simulink model "Tetris"  (R2023a)
settings: Solver=VariableStepAuto  StartTime=0.0  StopTime=inf  RelTol=1e-3  EnableMultiTasking=on
libraries: Miscellaneous x183, Byte_Multiplexers_Lib x77, Tetris_Lib x34, simulink_extras x11, Counters_Lib x7, Arithmetic_Operations_Lib x5, Word_Multiplexers_Lib x5, Decoders_Lib x4, Memory_Blocks_Lib x3, Bit_Multiplexers_Lib x2, dspobslib x1
(part 3 of 3)

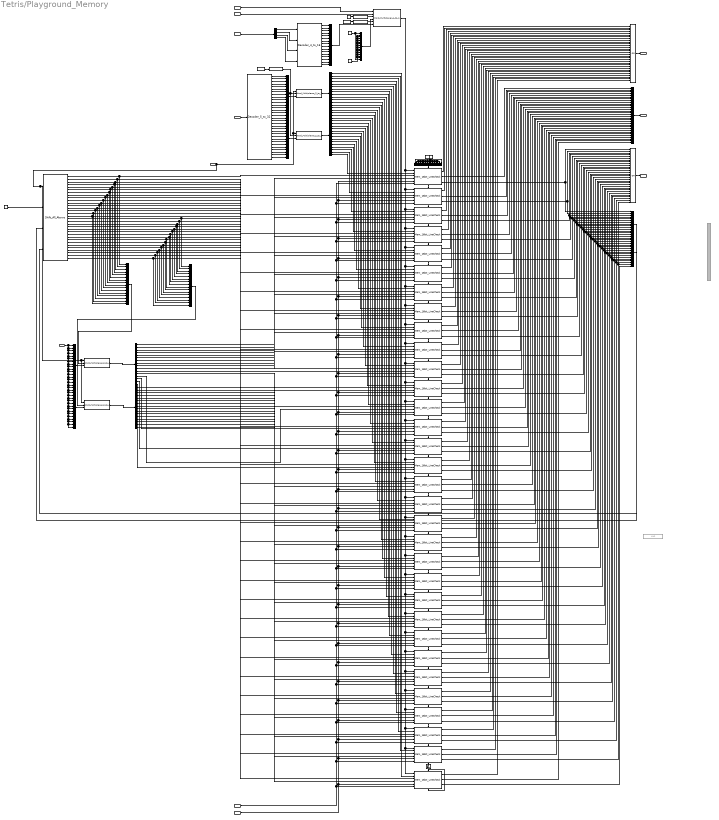
== system Tetris/Playground_Memory ==
  Sel_X(1B) : Inport
  Sel_Y(1B) : Inport  Port=2
  RowAccessUp(1b) : Inport  Port=3
  RowAccessDn(1b) : Inport  Port=4
  Write(1b) : Inport  Port=5
  Shift(1b) : Inport  Port=6
  Data(1b) : Inport  Port=7
  Clk : Inport  Port=8  OutDataTypeStr=boolean
  Bus Creator{1..2,4..6,8..13} (11 alike) : BusCreator  Inputs=16
  Bus Creator3 : BusCreator  Inputs=32
  Bus Creator7 : BusCreator  Commented=on  Inputs=32
  Bus Selector1 : BusSelector  OutputSignals=signal5,signal6,signal7,signal8
  Bus Selector{2..5} (4 alike) : BusSelector  OutputSignals=signal1,signal2,signal3,signal4,signal5,signal6,signal7,signal8,signal9,signal10,signal11,signal12,signal13,signal14,signal15,signal16
  Decoder_4_to_16 : Decoders_Lib/Decoders_Lib/Decoder_4_to_16  SystemSampleTime=-1  VariantActivationTime=update diagram  Latency=0  AutoFrameSizeCalculation=off
  Decoder_5_to_32 : Decoders_Lib/Decoders_Lib/Decoder_5_to_32  SystemSampleTime=-1  VariantActivationTime=update diagram  Latency=0  AutoFrameSizeCalculation=off
  Logical Operator1 : Logic  Operator=OR  Inputs=32  IconShape=distinctive  AllPortsSameDT=off  OutDataTypeStr=boolean
  Logical Operator2 : Logic  Commented=on  Inputs=12  IconShape=distinctive  AllPortsSameDT=off  OutDataTypeStr=boolean
  Logical Operator3 : Logic  Operator=OR  Inputs=31  IconShape=distinctive  AllPortsSameDT=off  OutDataTypeStr=boolean
  Mem_16bit_LineCheck{,1..31} (32 alike) : Tetris_Lib/Mem_16bit_LineCheck  SystemSampleTime=-1  VariantActivationTime=update diagram  Latency=0  AutoFrameSizeCalculation=off
      settings: PortSchema="{\"entries\":[{\"content\":{\"sides\":[{\"content\":{\"connectorIds\":[\"In1\",\"In2\",\"In3\",\"In4\",\"In5\",\"In6\"]},\"type\":\"ConnectorPlacement.EquallySpacedRectSide\",\"uuid\":\"8c2b0956-6f9d-4511-a90f-b568422ac059\"},{\"content\":{\"connectorIds\":[\"Out1\",\"Out2\",\"Out3\"],\"side\":\"RIGHT\"},\"type\":\"ConnectorPlacement.EquallySpacedRectSide\",\"uuid\":\"f2746d35-82bb-4709-925e-ccfde81ba195\"},{\"content\":{\"connectorIds\":[\"In7\"],\"side\":\"TOP\"},\"type\":\"ConnectorPlacement.EquallySpacedRectSide\",\"uuid\":\"2c21dbc3-5fbd-4074-80c1-0ed6354c6907\"},{\"content\":{\"connectorIds\":[\"Out4\"],\"side\":\"BOTTOM\"},\"type\":\"ConnectorPlacement.EquallySpacedRectSide\",\"uuid\":\"e35f839b-c525-4d99-8eb1-36043d411746\"}]},\"type\":\"ConnectorPlacement.EquallySpacedConnector\",\"uuid\":\"65dd92b9-0be0-4546-ad93-b6d7cfee0a19\"}],\"packageUris\":[\"http://schema.mathworks.com/mf0/Connector/R2020b\"],\"version\":\"1.0\"}"
  None1 : Constant  Value=0  OutDataTypeStr=boolean
  None2 : Constant  Value=0  OutDataTypeStr=boolean
  None3 : Constant  Value=0  OutDataTypeStr=boolean
  None4 : Constant  OutDataTypeStr=boolean
  NotUsed : Constant  Value=0  OutDataTypeStr=uint16
  SelectAllColumns : Constant  Value=65535  OutDataTypeStr=uint16
  SelectAllRows : Constant  Value=65535  OutDataTypeStr=uint16
  SelectInnerColumns : Constant  OutDataTypeStr=boolean
  Shift_All_Above : Tetris_Lib/Shift_All_Above  SystemSampleTime=-1  VariantActivationTime=update diagram  Latency=0  AutoFrameSizeCalculation=off
  Terminator : Terminator
  Word_Multiplexer_2_to_{1..4} (4 alike) : Word_Multiplexers_Lib/Word_Multiplexers_Lib/Word_Multiplexer_2_to_1  SystemSampleTime=-1  VariantActivationTime=update diagram  Latency=0  AutoFrameSizeCalculation=off
  Word_Multiplexer_4_to_1 : Word_Multiplexers_Lib/Word_Multiplexers_Lib/Word_Multiplexer_4_to_1  SystemSampleTime=-1  VariantActivationTime=update diagram  Latency=0  AutoFrameSizeCalculation=off
  uint_to_bus : Miscellaneous/uint_to_bus  SystemSampleTime=-1  VariantActivationTime=update diagram  Latency=0  AutoFrameSizeCalculation=off
  uint_to_bus1 : Miscellaneous/uint_to_bus  SystemSampleTime=-1  VariantActivationTime=update diagram  Latency=0  AutoFrameSizeCalculation=off
  uint_to_bus2 : Miscellaneous/uint_to_bus  SystemSampleTime=-1  VariantActivationTime=update diagram  Latency=0  AutoFrameSizeCalculation=off
  Video(32x16b) : Outport
  PixelOut(1b) : Outport  Port=2
  LineDone(1b) : Outport  Port=3
  wires:
  Bus Selector1/1 -> Decoder_4_to_16/1  "<signal5>"
  Bus Selector1/2 -> Decoder_4_to_16/2  "<signal6>"
  Bus Selector1/3 -> Decoder_4_to_16/3  "<signal7>"
  Bus Selector1/4 -> Decoder_4_to_16/4  "<signal8>"
  Sel_X(1B)/1 -> Bus Selector1/1
  Sel_Y(1B)/1 -> Decoder_5_to_32/1
  Bus Selector3/16 -> Mem_16bit_LineCheck31/2  "<signal16>"
  Bus Selector3/15 -> Mem_16bit_LineCheck30/2  "<signal15>"
  Bus Selector3/14 -> Mem_16bit_LineCheck29/2  "<signal14>"
  Bus Selector3/13 -> Mem_16bit_LineCheck28/2  "<signal13>"
  Bus Selector3/12 -> Mem_16bit_LineCheck27/2  "<signal12>"
  Bus Selector3/11 -> Mem_16bit_LineCheck26/2  "<signal11>"
  Bus Selector3/10 -> Mem_16bit_LineCheck25/2  "<signal10>"
  Bus Selector3/9 -> Mem_16bit_LineCheck24/2  "<signal9>"
  Bus Selector3/8 -> Mem_16bit_LineCheck23/2  "<signal8>"
  Bus Selector3/7 -> Mem_16bit_LineCheck22/2  "<signal7>"
  Bus Selector3/6 -> Mem_16bit_LineCheck21/2  "<signal6>"
  Bus Selector3/5 -> Mem_16bit_LineCheck20/2  "<signal5>"
  Bus Selector3/4 -> Mem_16bit_LineCheck19/2  "<signal4>"
  Bus Selector3/3 -> Mem_16bit_LineCheck18/2  "<signal3>"
  Bus Selector3/2 -> Mem_16bit_LineCheck17/2  "<signal2>"
  Bus Selector3/1 -> Mem_16bit_LineCheck16/2  "<signal1>"
  Bus Selector2/16 -> Mem_16bit_LineCheck15/2  "<signal16>"
  Bus Selector2/15 -> Mem_16bit_LineCheck14/2  "<signal15>"
  Bus Selector2/14 -> Mem_16bit_LineCheck13/2  "<signal14>"
  Bus Selector2/13 -> Mem_16bit_LineCheck12/2  "<signal13>"
  Bus Selector2/12 -> Mem_16bit_LineCheck11/2  "<signal12>"
  Bus Selector2/11 -> Mem_16bit_LineCheck10/2  "<signal11>"
  Bus Selector2/10 -> Mem_16bit_LineCheck9/2  "<signal10>"
  Bus Selector2/9 -> Mem_16bit_LineCheck8/2  "<signal9>"
  Bus Selector2/8 -> Mem_16bit_LineCheck7/2  "<signal8>"
  Bus Selector2/7 -> Mem_16bit_LineCheck6/2  "<signal7>"
  Bus Selector2/6 -> Mem_16bit_LineCheck5/2  "<signal6>"
  Bus Selector2/5 -> Mem_16bit_LineCheck4/2  "<signal5>"
  Bus Selector2/4 -> Mem_16bit_LineCheck3/2  "<signal4>"
  Bus Selector2/3 -> Mem_16bit_LineCheck2/2  "<signal3>"
  Bus Selector2/2 -> Mem_16bit_LineCheck1/2  "<signal2>"
  Bus Selector2/1 -> Mem_16bit_LineCheck/2  "<signal1>"
  Data(1b)/1 -> Mem_16bit_LineCheck31/5, Mem_16bit_LineCheck30/5, Mem_16bit_LineCheck29/5, Mem_16bit_LineCheck28/5, Mem_16bit_LineCheck27/5, Mem_16bit_LineCheck26/5, Mem_16bit_LineCheck25/5, Mem_16bit_LineCheck24/5, Mem_16bit_LineCheck23/5, Mem_16bit_LineCheck22/5, Mem_16bit_LineCheck21/5, Mem_16bit_LineCheck20/5, Mem_16bit_LineCheck19/5, Mem_16bit_LineCheck18/5, Mem_16bit_LineCheck17/5, Mem_16bit_LineCheck16/5, Mem_16bit_LineCheck15/5, Mem_16bit_LineCheck14/5, Mem_16bit_LineCheck13/5, Mem_16bit_LineCheck12/5, Mem_16bit_LineCheck11/5, Mem_16bit_LineCheck10/5, Mem_16bit_LineCheck9/5, Mem_16bit_LineCheck8/5, Mem_16bit_LineCheck7/5, Mem_16bit_LineCheck6/5, Mem_16bit_LineCheck5/5, Mem_16bit_LineCheck4/5, Mem_16bit_LineCheck3/5, Mem_16bit_LineCheck2/5, Mem_16bit_LineCheck1/5, Mem_16bit_LineCheck/5
  Clk/1 -> Mem_16bit_LineCheck31/6, Mem_16bit_LineCheck30/6, Mem_16bit_LineCheck29/6, Mem_16bit_LineCheck28/6, Mem_16bit_LineCheck27/6, Mem_16bit_LineCheck26/6, Mem_16bit_LineCheck25/6, Mem_16bit_LineCheck24/6, Mem_16bit_LineCheck23/6, Mem_16bit_LineCheck22/6, Mem_16bit_LineCheck21/6, Mem_16bit_LineCheck20/6, Mem_16bit_LineCheck19/6, Mem_16bit_LineCheck18/6, Mem_16bit_LineCheck17/6, Mem_16bit_LineCheck16/6, Mem_16bit_LineCheck15/6, Mem_16bit_LineCheck14/6, Mem_16bit_LineCheck13/6, Mem_16bit_LineCheck12/6, Mem_16bit_LineCheck11/6, Mem_16bit_LineCheck10/6, Mem_16bit_LineCheck9/6, Mem_16bit_LineCheck8/6, Mem_16bit_LineCheck7/6, Mem_16bit_LineCheck6/6, Mem_16bit_LineCheck5/6, Mem_16bit_LineCheck4/6, Mem_16bit_LineCheck3/6, Mem_16bit_LineCheck2/6, Mem_16bit_LineCheck1/6, Mem_16bit_LineCheck/6
  Mem_16bit_LineCheck31/2 -> Bus Creator3/1
  Mem_16bit_LineCheck30/2 -> Bus Creator3/2
  Mem_16bit_LineCheck29/2 -> Bus Creator3/3
  Mem_16bit_LineCheck28/2 -> Bus Creator3/4
  Mem_16bit_LineCheck27/2 -> Bus Creator3/5
  Mem_16bit_LineCheck26/2 -> Bus Creator3/6
  Mem_16bit_LineCheck25/2 -> Bus Creator3/7
  Mem_16bit_LineCheck24/2 -> Bus Creator3/8
  Mem_16bit_LineCheck23/2 -> Bus Creator3/9
  Mem_16bit_LineCheck22/2 -> Bus Creator3/10
  Mem_16bit_LineCheck21/2 -> Bus Creator3/11
  Mem_16bit_LineCheck20/2 -> Bus Creator3/12
  Mem_16bit_LineCheck19/2 -> Bus Creator3/13
  Mem_16bit_LineCheck18/2 -> Bus Creator3/14
  Mem_16bit_LineCheck17/2 -> Bus Creator3/15
  Mem_16bit_LineCheck16/2 -> Bus Creator3/16
  Mem_16bit_LineCheck15/2 -> Bus Creator3/17
  Mem_16bit_LineCheck14/2 -> Bus Creator3/18
  Mem_16bit_LineCheck13/2 -> Bus Creator3/19
  Mem_16bit_LineCheck12/2 -> Bus Creator3/20
  Mem_16bit_LineCheck11/2 -> Bus Creator3/21
  Mem_16bit_LineCheck10/2 -> Bus Creator3/22
  Mem_16bit_LineCheck9/2 -> Bus Creator3/23
  Mem_16bit_LineCheck8/2 -> Bus Creator3/24
  Mem_16bit_LineCheck7/2 -> Bus Creator3/25
  Mem_16bit_LineCheck6/2 -> Bus Creator3/26
  Mem_16bit_LineCheck5/2 -> Bus Creator3/27
  Mem_16bit_LineCheck4/2 -> Bus Creator3/28
  Mem_16bit_LineCheck3/2 -> Bus Creator3/29
  Mem_16bit_LineCheck2/2 -> Bus Creator3/30
  Mem_16bit_LineCheck1/2 -> Bus Creator3/31
  Mem_16bit_LineCheck/2 -> Bus Creator3/32
  Mem_16bit_LineCheck31/1 -> Logical Operator1/1
  Mem_16bit_LineCheck30/1 -> Logical Operator1/2
  Mem_16bit_LineCheck29/1 -> Logical Operator1/3
  Mem_16bit_LineCheck28/1 -> Logical Operator1/4
  Mem_16bit_LineCheck27/1 -> Logical Operator1/5
  Mem_16bit_LineCheck26/1 -> Logical Operator1/6
  Mem_16bit_LineCheck25/1 -> Logical Operator1/7
  Mem_16bit_LineCheck24/1 -> Logical Operator1/8
  Mem_16bit_LineCheck23/1 -> Logical Operator1/9
  Mem_16bit_LineCheck22/1 -> Logical Operator1/10
  Mem_16bit_LineCheck21/1 -> Logical Operator1/11
  Mem_16bit_LineCheck20/1 -> Logical Operator1/12
  Mem_16bit_LineCheck19/1 -> Logical Operator1/13
  Mem_16bit_LineCheck18/1 -> Logical Operator1/14
  Mem_16bit_LineCheck17/1 -> Logical Operator1/15
  Mem_16bit_LineCheck16/1 -> Logical Operator1/16
  Mem_16bit_LineCheck15/1 -> Logical Operator1/17
  Mem_16bit_LineCheck14/1 -> Logical Operator1/18
  Mem_16bit_LineCheck13/1 -> Logical Operator1/19
  Mem_16bit_LineCheck12/1 -> Logical Operator1/20
  Mem_16bit_LineCheck11/1 -> Logical Operator1/21
  Mem_16bit_LineCheck10/1 -> Logical Operator1/22
  Mem_16bit_LineCheck9/1 -> Logical Operator1/23
  Mem_16bit_LineCheck8/1 -> Logical Operator1/24
  Mem_16bit_LineCheck7/1 -> Logical Operator1/25
  Mem_16bit_LineCheck6/1 -> Logical Operator1/26
  Mem_16bit_LineCheck5/1 -> Logical Operator1/27
  Mem_16bit_LineCheck4/1 -> Logical Operator1/28
  Mem_16bit_LineCheck3/1 -> Logical Operator1/29
  Mem_16bit_LineCheck2/1 -> Logical Operator1/30
  Mem_16bit_LineCheck1/1 -> Logical Operator1/31
  Mem_16bit_LineCheck/1 -> Logical Operator1/32
  Bus Creator3/1 -> Video(32x16b)/1
  Logical Operator1/1 -> PixelOut(1b)/1
  RowAccessUp(1b)/1 -> Word_Multiplexer_4_to_1/2
  Bus Creator1/1 -> Word_Multiplexer_4_to_1/6
  Decoder_4_to_16/1 -> Bus Creator1/1
  Decoder_4_to_16/2 -> Bus Creator1/2
  Decoder_4_to_16/3 -> Bus Creator1/3
  Decoder_4_to_16/4 -> Bus Creator1/4
  Decoder_4_to_16/5 -> Bus Creator1/5
  Decoder_4_to_16/6 -> Bus Creator1/6
  Decoder_4_to_16/7 -> Bus Creator1/7
  Decoder_4_to_16/8 -> Bus Creator1/8
  Decoder_4_to_16/9 -> Bus Creator1/9
  Decoder_4_to_16/10 -> Bus Creator1/10
  Decoder_4_to_16/11 -> Bus Creator1/11
  Decoder_4_to_16/12 -> Bus Creator1/12
  Decoder_4_to_16/13 -> Bus Creator1/13
  Decoder_4_to_16/14 -> Bus Creator1/14
  Decoder_4_to_16/15 -> Bus Creator1/15
  Decoder_4_to_16/16 -> Bus Creator1/16
  Word_Multiplexer_4_to_1/1 -> Mem_16bit_LineCheck/1, Mem_16bit_LineCheck1/1, Mem_16bit_LineCheck2/1, Mem_16bit_LineCheck3/1, Mem_16bit_LineCheck4/1, Mem_16bit_LineCheck5/1, Mem_16bit_LineCheck6/1, Mem_16bit_LineCheck7/1, Mem_16bit_LineCheck8/1, Mem_16bit_LineCheck9/1, Mem_16bit_LineCheck10/1, Mem_16bit_LineCheck11/1, Mem_16bit_LineCheck12/1, Mem_16bit_LineCheck13/1, Mem_16bit_LineCheck14/1, Mem_16bit_LineCheck15/1, Mem_16bit_LineCheck16/1, Mem_16bit_LineCheck17/1, Mem_16bit_LineCheck18/1, Mem_16bit_LineCheck19/1, Mem_16bit_LineCheck20/1, Mem_16bit_LineCheck21/1, Mem_16bit_LineCheck22/1, Mem_16bit_LineCheck23/1, Mem_16bit_LineCheck24/1, Mem_16bit_LineCheck25/1, Mem_16bit_LineCheck26/1, Mem_16bit_LineCheck27/1, Mem_16bit_LineCheck28/1, Mem_16bit_LineCheck29/1, Mem_16bit_LineCheck30/1, Mem_16bit_LineCheck31/1
  Mem_16bit_LineCheck2/4 -> Mem_16bit_LineCheck1/7
  Mem_16bit_LineCheck1/4 -> Terminator/1
  Bus Creator2/1 -> Mem_16bit_LineCheck31/7
  Mem_16bit_LineCheck/4 -> Mem_16bit_LineCheck/7
  SelectInnerColumns/1 -> Bus Creator4/2, Bus Creator4/3, Bus Creator4/4, Bus Creator4/5, Bus Creator4/6, Bus Creator4/7, Bus Creator4/8, Bus Creator4/9, Bus Creator4/10, Bus Creator4/11, Bus Creator4/12, Bus Creator4/13, Bus Creator4/14, Bus Creator4/15
  None3/1 -> Bus Creator4/16, Bus Creator4/1
  Bus Creator4/1 -> Word_Multiplexer_4_to_1/4
  RowAccessDn(1b)/1 -> Word_Multiplexer_4_to_1/1
  uint_to_bus/1 -> Word_Multiplexer_4_to_1/3
  NotUsed/1 -> uint_to_bus/1
  SelectAllColumns/1 -> uint_to_bus1/1
  uint_to_bus1/1 -> Word_Multiplexer_4_to_1/5
  None4/1 -> Bus Creator2/16, Bus Creator2/1
  Decoder_5_to_32/18 -> Bus Creator5/2
  Decoder_5_to_32/19 -> Bus Creator5/3
  Decoder_5_to_32/20 -> Bus Creator5/4
  Decoder_5_to_32/21 -> Bus Creator5/5
  Decoder_5_to_32/22 -> Bus Creator5/6
  Decoder_5_to_32/23 -> Bus Creator5/7
  Decoder_5_to_32/24 -> Bus Creator5/8
  Decoder_5_to_32/25 -> Bus Creator5/9
  Decoder_5_to_32/26 -> Bus Creator5/10
  Decoder_5_to_32/27 -> Bus Creator5/11
  Decoder_5_to_32/28 -> Bus Creator5/12
  Decoder_5_to_32/29 -> Bus Creator5/13
  Decoder_5_to_32/30 -> Bus Creator5/14
  Decoder_5_to_32/31 -> Bus Creator5/15
  Decoder_5_to_32/32 -> Bus Creator5/16
  Decoder_5_to_32/1 -> Bus Creator6/1
  Decoder_5_to_32/2 -> Bus Creator6/2
  Decoder_5_to_32/3 -> Bus Creator6/3
  Decoder_5_to_32/4 -> Bus Creator6/4
  Decoder_5_to_32/5 -> Bus Creator6/5
  Decoder_5_to_32/6 -> Bus Creator6/6
  Decoder_5_to_32/7 -> Bus Creator6/7
  Decoder_5_to_32/8 -> Bus Creator6/8
  Decoder_5_to_32/9 -> Bus Creator6/9
  Decoder_5_to_32/10 -> Bus Creator6/10
  Decoder_5_to_32/11 -> Bus Creator6/11
  Decoder_5_to_32/12 -> Bus Creator6/12
  Decoder_5_to_32/13 -> Bus Creator6/13
  Decoder_5_to_32/14 -> Bus Creator6/14
  Decoder_5_to_32/15 -> Bus Creator6/15
  Decoder_5_to_32/16 -> Bus Creator6/16
  Decoder_5_to_32/17 -> Bus Creator5/1
  Bus Creator6/1 -> Word_Multiplexer_2_to_1/3
  Bus Creator5/1 -> Word_Multiplexer_2_to_2/3
  Word_Multiplexer_2_to_1/1 -> Bus Selector2/1
  Word_Multiplexer_2_to_2/1 -> Bus Selector3/1
  uint_to_bus2/1 -> Word_Multiplexer_2_to_2/2, Word_Multiplexer_2_to_1/2
  SelectAllRows/1 -> uint_to_bus2/1
  Mem_16bit_LineCheck4/4 -> Mem_16bit_LineCheck3/7
  Mem_16bit_LineCheck5/4 -> Mem_16bit_LineCheck4/7
  Mem_16bit_LineCheck6/4 -> Mem_16bit_LineCheck5/7
  Mem_16bit_LineCheck7/4 -> Mem_16bit_LineCheck6/7
  Mem_16bit_LineCheck8/4 -> Mem_16bit_LineCheck7/7
  Mem_16bit_LineCheck9/4 -> Mem_16bit_LineCheck8/7
  Mem_16bit_LineCheck10/4 -> Mem_16bit_LineCheck9/7
  Mem_16bit_LineCheck11/4 -> Mem_16bit_LineCheck10/7
  Mem_16bit_LineCheck12/4 -> Mem_16bit_LineCheck11/7
  Mem_16bit_LineCheck13/4 -> Mem_16bit_LineCheck12/7
  Mem_16bit_LineCheck14/4 -> Mem_16bit_LineCheck13/7
  Mem_16bit_LineCheck15/4 -> Mem_16bit_LineCheck14/7
  Mem_16bit_LineCheck16/4 -> Mem_16bit_LineCheck15/7
  Mem_16bit_LineCheck17/4 -> Mem_16bit_LineCheck16/7
  Mem_16bit_LineCheck18/4 -> Mem_16bit_LineCheck17/7
  Mem_16bit_LineCheck19/4 -> Mem_16bit_LineCheck18/7
  Mem_16bit_LineCheck20/4 -> Mem_16bit_LineCheck19/7
  Mem_16bit_LineCheck21/4 -> Mem_16bit_LineCheck20/7
  Mem_16bit_LineCheck22/4 -> Mem_16bit_LineCheck21/7
  Mem_16bit_LineCheck23/4 -> Mem_16bit_LineCheck22/7
  Mem_16bit_LineCheck24/4 -> Mem_16bit_LineCheck23/7
  Mem_16bit_LineCheck25/4 -> Mem_16bit_LineCheck24/7
  Mem_16bit_LineCheck26/4 -> Mem_16bit_LineCheck25/7
  Mem_16bit_LineCheck27/4 -> Mem_16bit_LineCheck26/7
  Mem_16bit_LineCheck28/4 -> Mem_16bit_LineCheck27/7
  Mem_16bit_LineCheck29/4 -> Mem_16bit_LineCheck28/7
  Mem_16bit_LineCheck30/4 -> Mem_16bit_LineCheck29/7
  Mem_16bit_LineCheck31/4 -> Mem_16bit_LineCheck30/7
  Mem_16bit_LineCheck3/4 -> Mem_16bit_LineCheck2/7
  Mem_16bit_LineCheck31/3 -> Bus Creator10/1, Logical Operator3/1
  Mem_16bit_LineCheck30/3 -> Bus Creator10/2, Logical Operator3/2
  Mem_16bit_LineCheck29/3 -> Bus Creator10/3, Logical Operator3/3
  Mem_16bit_LineCheck28/3 -> Bus Creator10/4, Logical Operator3/4
  Mem_16bit_LineCheck27/3 -> Bus Creator10/5, Logical Operator3/5
  Mem_16bit_LineCheck26/3 -> Bus Creator10/6, Logical Operator3/6
  Mem_16bit_LineCheck25/3 -> Bus Creator10/7, Logical Operator3/7
  Mem_16bit_LineCheck24/3 -> Bus Creator10/8, Logical Operator3/8
  Mem_16bit_LineCheck22/3 -> Bus Creator10/10, Logical Operator3/10
  Mem_16bit_LineCheck21/3 -> Bus Creator10/11, Logical Operator3/11
  Mem_16bit_LineCheck20/3 -> Bus Creator10/12, Logical Operator3/12
  Mem_16bit_LineCheck19/3 -> Bus Creator10/13, Logical Operator3/13
  Mem_16bit_LineCheck18/3 -> Bus Creator10/14, Logical Operator3/14
  Mem_16bit_LineCheck17/3 -> Bus Creator10/15, Logical Operator3/15
  Mem_16bit_LineCheck16/3 -> Bus Creator10/16, Logical Operator3/16
  Mem_16bit_LineCheck15/3 -> Bus Creator11/1, Logical Operator3/17
  Mem_16bit_LineCheck14/3 -> Bus Creator11/2, Logical Operator3/18
  Mem_16bit_LineCheck13/3 -> Bus Creator11/3, Logical Operator3/19
  Mem_16bit_LineCheck12/3 -> Bus Creator11/4, Logical Operator3/20
  Mem_16bit_LineCheck11/3 -> Bus Creator11/5, Logical Operator3/21
  Mem_16bit_LineCheck10/3 -> Bus Creator11/6, Logical Operator3/22
  Mem_16bit_LineCheck9/3 -> Bus Creator11/7, Logical Operator3/23
  Mem_16bit_LineCheck8/3 -> Bus Creator11/8, Logical Operator3/24
  Mem_16bit_LineCheck7/3 -> Bus Creator11/9, Logical Operator3/25
  Mem_16bit_LineCheck6/3 -> Bus Creator11/10, Logical Operator3/26
  Mem_16bit_LineCheck5/3 -> Bus Creator11/11, Logical Operator3/27
  Mem_16bit_LineCheck4/3 -> Bus Creator11/12, Logical Operator3/28
  Mem_16bit_LineCheck3/3 -> Bus Creator11/13, Logical Operator3/29
  Mem_16bit_LineCheck2/3 -> Bus Creator11/14, Logical Operator3/30
  Mem_16bit_LineCheck1/3 -> Bus Creator11/15, Logical Operator3/31
  Bus Creator10/1 -> Shift_All_Above/3
  Shift_All_Above/1 -> Bus Creator12/1, Mem_16bit_LineCheck31/3
  Shift_All_Above/2 -> Bus Creator12/2, Mem_16bit_LineCheck30/3
  Shift_All_Above/3 -> Bus Creator12/3, Mem_16bit_LineCheck29/3
  Shift_All_Above/4 -> Bus Creator12/4, Mem_16bit_LineCheck28/3
  Shift_All_Above/5 -> Bus Creator12/5, Mem_16bit_LineCheck27/3
  Shift_All_Above/6 -> Bus Creator12/6, Mem_16bit_LineCheck26/3
  Shift_All_Above/7 -> Bus Creator12/7, Mem_16bit_LineCheck25/3
  Shift_All_Above/8 -> Bus Creator12/8, Mem_16bit_LineCheck24/3
  Shift_All_Above/9 -> Bus Creator12/9, Mem_16bit_LineCheck23/3
  Shift_All_Above/10 -> Bus Creator12/10, Mem_16bit_LineCheck22/3
  Shift_All_Above/11 -> Bus Creator12/11, Mem_16bit_LineCheck21/3
  Shift_All_Above/12 -> Bus Creator12/12, Mem_16bit_LineCheck20/3
  Shift_All_Above/13 -> Bus Creator12/13, Mem_16bit_LineCheck19/3
  Shift_All_Above/14 -> Bus Creator12/14, Mem_16bit_LineCheck18/3
  Shift_All_Above/15 -> Bus Creator12/15, Mem_16bit_LineCheck17/3
  Shift_All_Above/16 -> Bus Creator12/16, Mem_16bit_LineCheck16/3
  Shift_All_Above/17 -> Bus Creator13/1, Mem_16bit_LineCheck15/3
  Shift_All_Above/18 -> Bus Creator13/2, Mem_16bit_LineCheck14/3
  Shift_All_Above/19 -> Bus Creator13/3, Mem_16bit_LineCheck13/3
  Shift_All_Above/20 -> Bus Creator13/4, Mem_16bit_LineCheck12/3
  Shift_All_Above/21 -> Bus Creator13/5, Mem_16bit_LineCheck11/3
  Shift_All_Above/22 -> Bus Creator13/6, Mem_16bit_LineCheck10/3
  Shift_All_Above/23 -> Bus Creator13/7, Mem_16bit_LineCheck9/3
  Shift_All_Above/24 -> Bus Creator13/8, Mem_16bit_LineCheck8/3
  Shift_All_Above/25 -> Bus Creator13/9, Mem_16bit_LineCheck7/3
  Shift_All_Above/26 -> Bus Creator13/10, Mem_16bit_LineCheck6/3
  Shift_All_Above/27 -> Bus Creator13/11, Mem_16bit_LineCheck5/3
  Shift_All_Above/28 -> Bus Creator13/12, Mem_16bit_LineCheck4/3
  Shift_All_Above/29 -> Bus Creator13/13, Mem_16bit_LineCheck3/3
  Shift_All_Above/30 -> Bus Creator13/14, Mem_16bit_LineCheck2/3
  Shift_All_Above/31 -> Bus Creator13/15, Mem_16bit_LineCheck1/3
  Shift(1b)/1 -> Shift_All_Above/1, Word_Multiplexer_2_to_3/1, Word_Multiplexer_2_to_4/1, Word_Multiplexer_2_to_2/1, Word_Multiplexer_2_to_1/1
  Mem_16bit_LineCheck23/3 -> Bus Creator10/9, Logical Operator3/9
  Logical Operator3/1 -> LineDone(1b)/1
  Mem_16bit_LineCheck/3 -> Bus Creator11/16
  Shift_All_Above/32 -> Bus Creator13/16, Mem_16bit_LineCheck/3
  Bus Creator8/1 -> Word_Multiplexer_2_to_3/3
  Word_Multiplexer_2_to_3/1 -> Bus Selector4/1
  Bus Creator9/1 -> Word_Multiplexer_2_to_4/3
  Word_Multiplexer_2_to_4/1 -> Bus Selector5/1
  Write(1b)/1 -> Bus Creator8/2, Bus Creator8/3, Bus Creator8/4, Bus Creator8/5, Bus Creator8/6, Bus Creator8/7, Bus Creator8/8, Bus Creator8/9, Bus Creator8/10, Bus Creator8/11, Bus Creator8/12, Bus Creator8/13, Bus Creator8/14, Bus Creator8/15, Bus Creator8/16, Bus Creator9/1, Bus Creator9/2, Bus Creator9/3, Bus Creator9/4, Bus Creator9/5, Bus Creator9/6, Bus Creator9/7, Bus Creator9/8, Bus Creator9/9, Bus Creator9/10, Bus Creator9/11, Bus Creator9/12, Bus Creator9/13, Bus Creator9/14, Bus Creator9/15, Bus Creator9/16, Bus Creator8/1
  Bus Selector4/1 -> Mem_16bit_LineCheck31/4  "<signal1>"
  Bus Selector4/2 -> Mem_16bit_LineCheck30/4  "<signal2>"
  Bus Selector4/3 -> Mem_16bit_LineCheck29/4  "<signal3>"
  Bus Selector4/4 -> Mem_16bit_LineCheck28/4  "<signal4>"
  Bus Selector4/5 -> Mem_16bit_LineCheck27/4  "<signal5>"
  Bus Selector4/6 -> Mem_16bit_LineCheck26/4  "<signal6>"
  Bus Selector4/7 -> Mem_16bit_LineCheck25/4  "<signal7>"
  Bus Selector4/8 -> Mem_16bit_LineCheck24/4  "<signal8>"
  Bus Selector4/9 -> Mem_16bit_LineCheck23/4  "<signal9>"
  Bus Selector4/10 -> Mem_16bit_LineCheck22/4  "<signal10>"
  Bus Selector4/11 -> Mem_16bit_LineCheck21/4  "<signal11>"
  Bus Selector4/12 -> Mem_16bit_LineCheck20/4  "<signal12>"
  Bus Selector4/13 -> Mem_16bit_LineCheck19/4  "<signal13>"
  Bus Selector4/14 -> Mem_16bit_LineCheck18/4  "<signal14>"
  Bus Selector4/15 -> Mem_16bit_LineCheck17/4  "<signal15>"
  Bus Selector4/16 -> Mem_16bit_LineCheck16/4  "<signal16>"
  Bus Selector5/1 -> Mem_16bit_LineCheck15/4  "<signal1>"
  Bus Selector5/2 -> Mem_16bit_LineCheck14/4  "<signal2>"
  Bus Selector5/3 -> Mem_16bit_LineCheck13/4  "<signal3>"
  Bus Selector5/4 -> Mem_16bit_LineCheck12/4  "<signal4>"
  Bus Selector5/5 -> Mem_16bit_LineCheck11/4  "<signal5>"
  Bus Selector5/6 -> Mem_16bit_LineCheck10/4  "<signal6>"
  Bus Selector5/7 -> Mem_16bit_LineCheck9/4  "<signal7>"
  Bus Selector5/8 -> Mem_16bit_LineCheck8/4  "<signal8>"
  Bus Selector5/9 -> Mem_16bit_LineCheck7/4  "<signal9>"
  Bus Selector5/10 -> Mem_16bit_LineCheck6/4  "<signal10>"
  Bus Selector5/11 -> Mem_16bit_LineCheck5/4  "<signal11>"
  Bus Selector5/12 -> Mem_16bit_LineCheck4/4  "<signal12>"
  Bus Selector5/13 -> Mem_16bit_LineCheck3/4  "<signal13>"
  Bus Selector5/14 -> Mem_16bit_LineCheck2/4  "<signal14>"
  Bus Selector5/15 -> Mem_16bit_LineCheck1/4  "<signal15>"
  Bus Selector5/16 -> Mem_16bit_LineCheck/4  "<signal16>"
  Bus Creator11/1 -> Shift_All_Above/4
  None2/1 -> Shift_All_Above/2
  Bus Creator12/1 -> Word_Multiplexer_2_to_3/2
  Bus Creator13/1 -> Word_Multiplexer_2_to_4/2
  None1/1 -> Bus Creator2/12, Bus Creator2/14, Bus Creator2/15, Bus Creator2/13, Bus Creator2/11, Bus Creator2/10, Bus Creator2/9, Bus Creator2/2, Bus Creator2/3, Bus Creator2/4, Bus Creator2/5, Bus Creator2/6, Bus Creator2/7, Bus Creator2/8

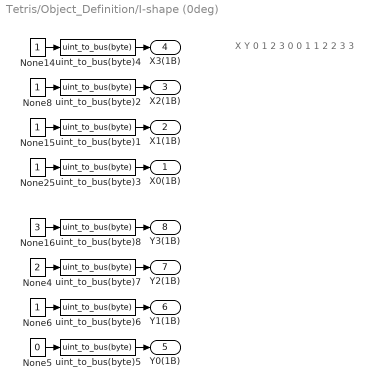
== system Tetris/Object_Definition/I-shape (0deg) ==
  note: X
      |
      | Y
      |
      | 0
      | 1
      | 2
      | 3
      |
      | 0
      |
      | 0
      |
      | 1
      |
      | 1
      |
      | 2
      |
      | 2
      |
      | 3
      |
      | 3
  None{6,8,14..15,25} (5 alike) : Constant  OutDataTypeStr=uint8
  None16 : Constant  Value=3  OutDataTypeStr=uint8
  None4 : Constant  Value=2  OutDataTypeStr=uint8
  None5 : Constant  Value=0  OutDataTypeStr=uint8
  uint_to_bus(byte){1..8} (8 alike) : Miscellaneous/uint_to_bus(byte)  SystemSampleTime=-1  VariantActivationTime=update diagram  Latency=0  AutoFrameSizeCalculation=off
  X0(1B) : Outport
  X1(1B) : Outport  Port=2
  X2(1B) : Outport  Port=3
  X3(1B) : Outport  Port=4
  Y0(1B) : Outport  Port=5
  Y1(1B) : Outport  Port=6
  Y2(1B) : Outport  Port=7
  Y3(1B) : Outport  Port=8
  wires:
  uint_to_bus(byte)4/1 -> X3(1B)/1
  None14/1 -> uint_to_bus(byte)4/1
  None25/1 -> uint_to_bus(byte)3/1
  None8/1 -> uint_to_bus(byte)2/1
  None15/1 -> uint_to_bus(byte)1/1
  uint_to_bus(byte)8/1 -> Y3(1B)/1
  uint_to_bus(byte)6/1 -> Y1(1B)/1
  None6/1 -> uint_to_bus(byte)6/1
  uint_to_bus(byte)7/1 -> Y2(1B)/1
  uint_to_bus(byte)5/1 -> Y0(1B)/1
  None16/1 -> uint_to_bus(byte)8/1
  None5/1 -> uint_to_bus(byte)5/1
  uint_to_bus(byte)1/1 -> X1(1B)/1
  uint_to_bus(byte)3/1 -> X0(1B)/1
  uint_to_bus(byte)2/1 -> X2(1B)/1
  None4/1 -> uint_to_bus(byte)7/1

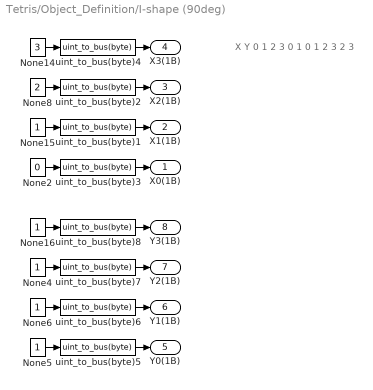
== system Tetris/Object_Definition/I-shape (90deg) ==
  note: X
      |
      | Y
      |
      | 0
      | 1
      | 2
      | 3
      |
      | 0
      |
      | 1
      | 0
      | 1
      | 2
      | 3
      |
      | 2
      |
      | 3
  None14 : Constant  Value=3  OutDataTypeStr=uint8
  None{4..6,15..16} (5 alike) : Constant  OutDataTypeStr=uint8
  None2 : Constant  Value=0  OutDataTypeStr=uint8
  None8 : Constant  Value=2  OutDataTypeStr=uint8
  uint_to_bus(byte){1..8} (8 alike) : Miscellaneous/uint_to_bus(byte)  SystemSampleTime=-1  VariantActivationTime=update diagram  Latency=0  AutoFrameSizeCalculation=off
  X0(1B) : Outport
  X1(1B) : Outport  Port=2
  X2(1B) : Outport  Port=3
  X3(1B) : Outport  Port=4
  Y0(1B) : Outport  Port=5
  Y1(1B) : Outport  Port=6
  Y2(1B) : Outport  Port=7
  Y3(1B) : Outport  Port=8
  wires:
  uint_to_bus(byte)8/1 -> Y3(1B)/1
  uint_to_bus(byte)2/1 -> X2(1B)/1
  None16/1 -> uint_to_bus(byte)8/1
  None4/1 -> uint_to_bus(byte)7/1
  None8/1 -> uint_to_bus(byte)2/1
  None15/1 -> uint_to_bus(byte)1/1
  None2/1 -> uint_to_bus(byte)3/1
  uint_to_bus(byte)1/1 -> X1(1B)/1
  uint_to_bus(byte)5/1 -> Y0(1B)/1
  None14/1 -> uint_to_bus(byte)4/1
  uint_to_bus(byte)7/1 -> Y2(1B)/1
  None6/1 -> uint_to_bus(byte)6/1
  uint_to_bus(byte)4/1 -> X3(1B)/1
  uint_to_bus(byte)3/1 -> X0(1B)/1
  uint_to_bus(byte)6/1 -> Y1(1B)/1
  None5/1 -> uint_to_bus(byte)5/1

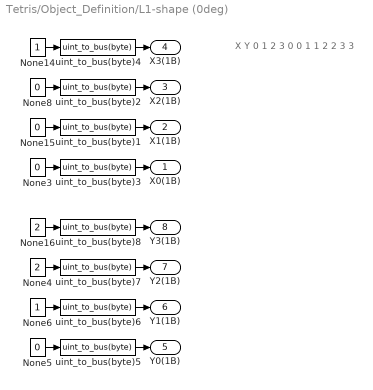
== system Tetris/Object_Definition/L1-shape (0deg) ==
  note: X
      |
      | Y
      |
      | 0
      | 1
      | 2
      | 3
      |
      | 0
      | 0
      |
      | 1
      | 1
      |
      | 2
      | 2
      | 3
      |
      | 3
  None14 : Constant  OutDataTypeStr=uint8
  None{3,5,8,15} (4 alike) : Constant  Value=0  OutDataTypeStr=uint8
  None16 : Constant  Value=2  OutDataTypeStr=uint8
  None4 : Constant  Value=2  OutDataTypeStr=uint8
  None6 : Constant  OutDataTypeStr=uint8
  uint_to_bus(byte){1..8} (8 alike) : Miscellaneous/uint_to_bus(byte)  SystemSampleTime=-1  VariantActivationTime=update diagram  Latency=0  AutoFrameSizeCalculation=off
  X0(1B) : Outport
  X1(1B) : Outport  Port=2
  X2(1B) : Outport  Port=3
  X3(1B) : Outport  Port=4
  Y0(1B) : Outport  Port=5
  Y1(1B) : Outport  Port=6
  Y2(1B) : Outport  Port=7
  Y3(1B) : Outport  Port=8
  wires:
  uint_to_bus(byte)1/1 -> X1(1B)/1
  uint_to_bus(byte)6/1 -> Y1(1B)/1
  None16/1 -> uint_to_bus(byte)8/1
  uint_to_bus(byte)8/1 -> Y3(1B)/1
  uint_to_bus(byte)7/1 -> Y2(1B)/1
  None4/1 -> uint_to_bus(byte)7/1
  uint_to_bus(byte)2/1 -> X2(1B)/1
  None8/1 -> uint_to_bus(byte)2/1
  None3/1 -> uint_to_bus(byte)3/1
  None5/1 -> uint_to_bus(byte)5/1
  uint_to_bus(byte)3/1 -> X0(1B)/1
  uint_to_bus(byte)5/1 -> Y0(1B)/1
  None6/1 -> uint_to_bus(byte)6/1
  None15/1 -> uint_to_bus(byte)1/1
  None14/1 -> uint_to_bus(byte)4/1
  uint_to_bus(byte)4/1 -> X3(1B)/1

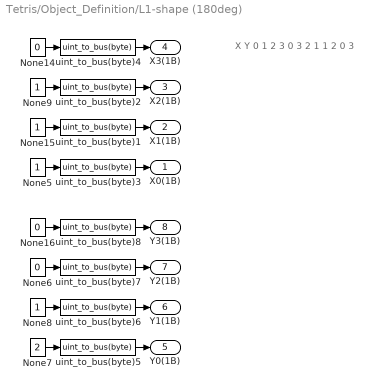
== system Tetris/Object_Definition/L1-shape (180deg) ==
  note: X
      |
      | Y
      |
      | 0
      | 1
      | 2
      | 3
      |
      | 0
      | 3
      | 2
      |
      | 1
      |
      | 1
      |
      | 2
      |
      | 0
      |
      | 3
  None14 : Constant  Value=0  OutDataTypeStr=uint8
  None{5,8..9,15} (4 alike) : Constant  OutDataTypeStr=uint8
  None16 : Constant  Value=0  OutDataTypeStr=uint8
  None6 : Constant  Value=0  OutDataTypeStr=uint8
  None7 : Constant  Value=2  OutDataTypeStr=uint8
  uint_to_bus(byte){1..8} (8 alike) : Miscellaneous/uint_to_bus(byte)  SystemSampleTime=-1  VariantActivationTime=update diagram  Latency=0  AutoFrameSizeCalculation=off
  X0(1B) : Outport
  X1(1B) : Outport  Port=2
  X2(1B) : Outport  Port=3
  X3(1B) : Outport  Port=4
  Y0(1B) : Outport  Port=5
  Y1(1B) : Outport  Port=6
  Y2(1B) : Outport  Port=7
  Y3(1B) : Outport  Port=8
  wires:
  uint_to_bus(byte)1/1 -> X1(1B)/1
  uint_to_bus(byte)6/1 -> Y1(1B)/1
  None16/1 -> uint_to_bus(byte)8/1
  uint_to_bus(byte)8/1 -> Y3(1B)/1
  uint_to_bus(byte)7/1 -> Y2(1B)/1
  None6/1 -> uint_to_bus(byte)7/1
  uint_to_bus(byte)2/1 -> X2(1B)/1
  None9/1 -> uint_to_bus(byte)2/1
  None5/1 -> uint_to_bus(byte)3/1
  None7/1 -> uint_to_bus(byte)5/1
  uint_to_bus(byte)3/1 -> X0(1B)/1
  uint_to_bus(byte)5/1 -> Y0(1B)/1
  None8/1 -> uint_to_bus(byte)6/1
  None15/1 -> uint_to_bus(byte)1/1
  None14/1 -> uint_to_bus(byte)4/1
  uint_to_bus(byte)4/1 -> X3(1B)/1

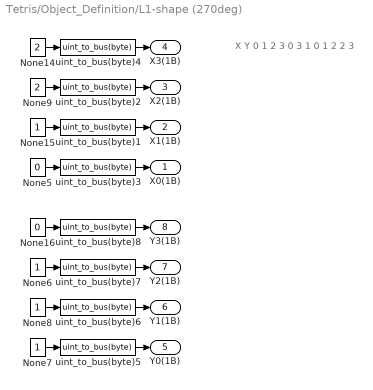
== system Tetris/Object_Definition/L1-shape (270deg) ==
  note: X
      |
      | Y
      |
      | 0
      | 1
      | 2
      | 3
      |
      | 0
      |
      | 3
      |
      | 1
      | 0
      | 1
      | 2
      |
      | 2
      |
      | 3
  None14 : Constant  Value=2  OutDataTypeStr=uint8
  None{6..8,15} (4 alike) : Constant  OutDataTypeStr=uint8
  None16 : Constant  Value=0  OutDataTypeStr=uint8
  None5 : Constant  Value=0  OutDataTypeStr=uint8
  None9 : Constant  Value=2  OutDataTypeStr=uint8
  uint_to_bus(byte){1..8} (8 alike) : Miscellaneous/uint_to_bus(byte)  SystemSampleTime=-1  VariantActivationTime=update diagram  Latency=0  AutoFrameSizeCalculation=off
  X0(1B) : Outport
  X1(1B) : Outport  Port=2
  X2(1B) : Outport  Port=3
  X3(1B) : Outport  Port=4
  Y0(1B) : Outport  Port=5
  Y1(1B) : Outport  Port=6
  Y2(1B) : Outport  Port=7
  Y3(1B) : Outport  Port=8
  wires:
  uint_to_bus(byte)1/1 -> X1(1B)/1
  uint_to_bus(byte)6/1 -> Y1(1B)/1
  None16/1 -> uint_to_bus(byte)8/1
  uint_to_bus(byte)8/1 -> Y3(1B)/1
  uint_to_bus(byte)7/1 -> Y2(1B)/1
  None6/1 -> uint_to_bus(byte)7/1
  uint_to_bus(byte)2/1 -> X2(1B)/1
  None9/1 -> uint_to_bus(byte)2/1
  None5/1 -> uint_to_bus(byte)3/1
  None7/1 -> uint_to_bus(byte)5/1
  uint_to_bus(byte)3/1 -> X0(1B)/1
  uint_to_bus(byte)5/1 -> Y0(1B)/1
  None8/1 -> uint_to_bus(byte)6/1
  None15/1 -> uint_to_bus(byte)1/1
  None14/1 -> uint_to_bus(byte)4/1
  uint_to_bus(byte)4/1 -> X3(1B)/1

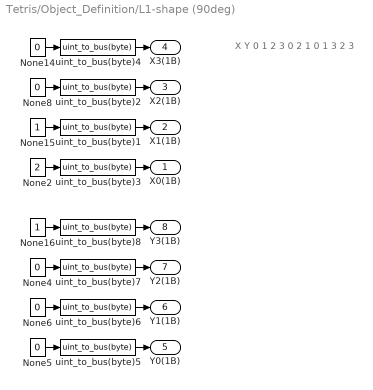
== system Tetris/Object_Definition/L1-shape (90deg) ==
  note: X
      |
      | Y
      |
      | 0
      | 1
      | 2
      | 3
      |
      | 0
      | 2
      | 1
      | 0
      |
      | 1
      | 3
      |
      | 2
      |
      | 3
  None{4..6,8,14} (5 alike) : Constant  Value=0  OutDataTypeStr=uint8
  None15 : Constant  OutDataTypeStr=uint8
  None16 : Constant  OutDataTypeStr=uint8
  None2 : Constant  Value=2  OutDataTypeStr=uint8
  uint_to_bus(byte){1..8} (8 alike) : Miscellaneous/uint_to_bus(byte)  SystemSampleTime=-1  VariantActivationTime=update diagram  Latency=0  AutoFrameSizeCalculation=off
  X0(1B) : Outport
  X1(1B) : Outport  Port=2
  X2(1B) : Outport  Port=3
  X3(1B) : Outport  Port=4
  Y0(1B) : Outport  Port=5
  Y1(1B) : Outport  Port=6
  Y2(1B) : Outport  Port=7
  Y3(1B) : Outport  Port=8
  wires:
  uint_to_bus(byte)1/1 -> X1(1B)/1
  uint_to_bus(byte)6/1 -> Y1(1B)/1
  None16/1 -> uint_to_bus(byte)8/1
  uint_to_bus(byte)8/1 -> Y3(1B)/1
  uint_to_bus(byte)7/1 -> Y2(1B)/1
  None4/1 -> uint_to_bus(byte)7/1
  uint_to_bus(byte)2/1 -> X2(1B)/1
  None8/1 -> uint_to_bus(byte)2/1
  None2/1 -> uint_to_bus(byte)3/1
  None5/1 -> uint_to_bus(byte)5/1
  uint_to_bus(byte)3/1 -> X0(1B)/1
  uint_to_bus(byte)5/1 -> Y0(1B)/1
  None6/1 -> uint_to_bus(byte)6/1
  None15/1 -> uint_to_bus(byte)1/1
  None14/1 -> uint_to_bus(byte)4/1
  uint_to_bus(byte)4/1 -> X3(1B)/1

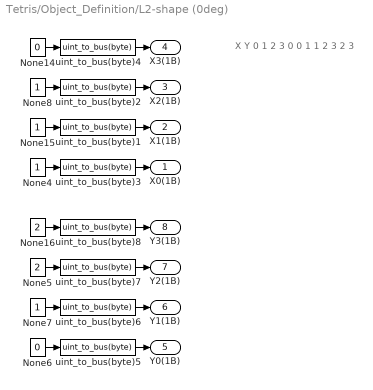
== system Tetris/Object_Definition/L2-shape (0deg) ==
  note: X
      |
      | Y
      |
      | 0
      | 1
      | 2
      | 3
      |
      | 0
      |
      | 0
      |
      | 1
      |
      | 1
      |
      | 2
      | 3
      | 2
      |
      | 3
  None14 : Constant  Value=0  OutDataTypeStr=uint8
  None{4,7..8,15} (4 alike) : Constant  OutDataTypeStr=uint8
  None16 : Constant  Value=2  OutDataTypeStr=uint8
  None5 : Constant  Value=2  OutDataTypeStr=uint8
  None6 : Constant  Value=0  OutDataTypeStr=uint8
  uint_to_bus(byte){1..8} (8 alike) : Miscellaneous/uint_to_bus(byte)  SystemSampleTime=-1  VariantActivationTime=update diagram  Latency=0  AutoFrameSizeCalculation=off
  X0(1B) : Outport
  X1(1B) : Outport  Port=2
  X2(1B) : Outport  Port=3
  X3(1B) : Outport  Port=4
  Y0(1B) : Outport  Port=5
  Y1(1B) : Outport  Port=6
  Y2(1B) : Outport  Port=7
  Y3(1B) : Outport  Port=8
  wires:
  uint_to_bus(byte)1/1 -> X1(1B)/1
  uint_to_bus(byte)6/1 -> Y1(1B)/1
  None16/1 -> uint_to_bus(byte)8/1
  uint_to_bus(byte)8/1 -> Y3(1B)/1
  uint_to_bus(byte)7/1 -> Y2(1B)/1
  None5/1 -> uint_to_bus(byte)7/1
  uint_to_bus(byte)2/1 -> X2(1B)/1
  None8/1 -> uint_to_bus(byte)2/1
  None4/1 -> uint_to_bus(byte)3/1
  None6/1 -> uint_to_bus(byte)5/1
  uint_to_bus(byte)3/1 -> X0(1B)/1
  uint_to_bus(byte)5/1 -> Y0(1B)/1
  None7/1 -> uint_to_bus(byte)6/1
  None15/1 -> uint_to_bus(byte)1/1
  None14/1 -> uint_to_bus(byte)4/1
  uint_to_bus(byte)4/1 -> X3(1B)/1

== system Tetris/Object_Definition/L2-shape (180deg) ==
  note: X
      |
      | Y
      |
      | 0
      | 1
      | 2
      | 3
      |
      | 0
      | 2
      | 3
      |
      | 1
      | 1
      |
      | 2
      | 0
      |
      | 3
  None14 : Constant  OutDataTypeStr=uint8
  None{3..4,8,15..16} (5 alike) : Constant  Value=0  OutDataTypeStr=uint8
  None5 : Constant  Value=2  OutDataTypeStr=uint8
  None6 : Constant  OutDataTypeStr=uint8
  uint_to_bus(byte){1..8} (8 alike) : Miscellaneous/uint_to_bus(byte)  SystemSampleTime=-1  VariantActivationTime=update diagram  Latency=0  AutoFrameSizeCalculation=off
  X0(1B) : Outport
  X1(1B) : Outport  Port=2
  X2(1B) : Outport  Port=3
  X3(1B) : Outport  Port=4
  Y0(1B) : Outport  Port=5
  Y1(1B) : Outport  Port=6
  Y2(1B) : Outport  Port=7
  Y3(1B) : Outport  Port=8
  wires:
  uint_to_bus(byte)1/1 -> X1(1B)/1
  uint_to_bus(byte)6/1 -> Y1(1B)/1
  None16/1 -> uint_to_bus(byte)8/1
  uint_to_bus(byte)8/1 -> Y3(1B)/1
  uint_to_bus(byte)7/1 -> Y2(1B)/1
  None4/1 -> uint_to_bus(byte)7/1
  uint_to_bus(byte)2/1 -> X2(1B)/1
  None8/1 -> uint_to_bus(byte)2/1
  None3/1 -> uint_to_bus(byte)3/1
  None5/1 -> uint_to_bus(byte)5/1
  uint_to_bus(byte)3/1 -> X0(1B)/1
  uint_to_bus(byte)5/1 -> Y0(1B)/1
  None6/1 -> uint_to_bus(byte)6/1
  None15/1 -> uint_to_bus(byte)1/1
  None14/1 -> uint_to_bus(byte)4/1
  uint_to_bus(byte)4/1 -> X3(1B)/1

== system Tetris/Object_Definition/L2-shape (270deg) ==
  note: X
      |
      | Y
      |
      | 0
      | 1
      | 2
      | 3
      |
      | 0
      | 0
      | 1
      | 2
      |
      | 1
      |
      | 3
      |
      | 2
      |
      | 3
  None14 : Constant  Value=2  OutDataTypeStr=uint8
  None15 : Constant  OutDataTypeStr=uint8
  None16 : Constant  OutDataTypeStr=uint8
  None{3..6} (4 alike) : Constant  Value=0  OutDataTypeStr=uint8
  None8 : Constant  Value=2  OutDataTypeStr=uint8
  uint_to_bus(byte){1..8} (8 alike) : Miscellaneous/uint_to_bus(byte)  SystemSampleTime=-1  VariantActivationTime=update diagram  Latency=0  AutoFrameSizeCalculation=off
  X0(1B) : Outport
  X1(1B) : Outport  Port=2
  X2(1B) : Outport  Port=3
  X3(1B) : Outport  Port=4
  Y0(1B) : Outport  Port=5
  Y1(1B) : Outport  Port=6
  Y2(1B) : Outport  Port=7
  Y3(1B) : Outport  Port=8
  wires:
  uint_to_bus(byte)1/1 -> X1(1B)/1
  uint_to_bus(byte)6/1 -> Y1(1B)/1
  None16/1 -> uint_to_bus(byte)8/1
  uint_to_bus(byte)8/1 -> Y3(1B)/1
  uint_to_bus(byte)7/1 -> Y2(1B)/1
  None4/1 -> uint_to_bus(byte)7/1
  uint_to_bus(byte)2/1 -> X2(1B)/1
  None8/1 -> uint_to_bus(byte)2/1
  None3/1 -> uint_to_bus(byte)3/1
  None5/1 -> uint_to_bus(byte)5/1
  uint_to_bus(byte)3/1 -> X0(1B)/1
  uint_to_bus(byte)5/1 -> Y0(1B)/1
  None6/1 -> uint_to_bus(byte)6/1
  None15/1 -> uint_to_bus(byte)1/1
  None14/1 -> uint_to_bus(byte)4/1
  uint_to_bus(byte)4/1 -> X3(1B)/1

== system Tetris/Object_Definition/L2-shape (90deg) ==
  note: X
      |
      | Y
      |
      | 0
      | 1
      | 2
      | 3
      |
      | 0
      | 3
      |
      | 1
      | 2
      | 1
      | 0
      |
      | 2
      |
      | 3
  None14 : Constant  Value=0  OutDataTypeStr=uint8
  None{5..7,15} (4 alike) : Constant  OutDataTypeStr=uint8
  None16 : Constant  Value=0  OutDataTypeStr=uint8
  None4 : Constant  Value=2  OutDataTypeStr=uint8
  None8 : Constant  Value=0  OutDataTypeStr=uint8
  uint_to_bus(byte){1..8} (8 alike) : Miscellaneous/uint_to_bus(byte)  SystemSampleTime=-1  VariantActivationTime=update diagram  Latency=0  AutoFrameSizeCalculation=off
  X0(1B) : Outport
  X1(1B) : Outport  Port=2
  X2(1B) : Outport  Port=3
  X3(1B) : Outport  Port=4
  Y0(1B) : Outport  Port=5
  Y1(1B) : Outport  Port=6
  Y2(1B) : Outport  Port=7
  Y3(1B) : Outport  Port=8
  wires:
  uint_to_bus(byte)1/1 -> X1(1B)/1
  uint_to_bus(byte)6/1 -> Y1(1B)/1
  None16/1 -> uint_to_bus(byte)8/1
  uint_to_bus(byte)8/1 -> Y3(1B)/1
  uint_to_bus(byte)7/1 -> Y2(1B)/1
  None5/1 -> uint_to_bus(byte)7/1
  uint_to_bus(byte)2/1 -> X2(1B)/1
  None8/1 -> uint_to_bus(byte)2/1
  None4/1 -> uint_to_bus(byte)3/1
  None6/1 -> uint_to_bus(byte)5/1
  uint_to_bus(byte)3/1 -> X0(1B)/1
  uint_to_bus(byte)5/1 -> Y0(1B)/1
  None7/1 -> uint_to_bus(byte)6/1
  None15/1 -> uint_to_bus(byte)1/1
  None14/1 -> uint_to_bus(byte)4/1
  uint_to_bus(byte)4/1 -> X3(1B)/1

== system Tetris/Object_Definition/O-shape ==
  note: X
      |
      | Y
      |
      | 0
      | 1
      | 2
      | 3
      |
      | 0
      | 0
      | 1
      |
      | 1
      | 2
      | 3
      |
      | 2
      |
      | 3
  None{1,14..16} (4 alike) : Constant  Value=0  OutDataTypeStr=uint8
  None{2..3,8,25} (4 alike) : Constant  OutDataTypeStr=uint8
  uint_to_bus(byte){1..8} (8 alike) : Miscellaneous/uint_to_bus(byte)  SystemSampleTime=-1  VariantActivationTime=update diagram  Latency=0  AutoFrameSizeCalculation=off
  X0(1B) : Outport
  X1(1B) : Outport  Port=2
  X2(1B) : Outport  Port=3
  X3(1B) : Outport  Port=4
  Y0(1B) : Outport  Port=5
  Y1(1B) : Outport  Port=6
  Y2(1B) : Outport  Port=7
  Y3(1B) : Outport  Port=8
  wires:
  uint_to_bus(byte)5/1 -> Y3(1B)/1
  uint_to_bus(byte)2/1 -> X1(1B)/1
  uint_to_bus(byte)6/1 -> Y2(1B)/1
  None15/1 -> uint_to_bus(byte)1/1
  uint_to_bus(byte)3/1 -> X3(1B)/1
  None25/1 -> uint_to_bus(byte)3/1
  None8/1 -> uint_to_bus(byte)2/1
  uint_to_bus(byte)4/1 -> X0(1B)/1
  uint_to_bus(byte)7/1 -> Y1(1B)/1
  None14/1 -> uint_to_bus(byte)4/1
  uint_to_bus(byte)1/1 -> X2(1B)/1
  uint_to_bus(byte)8/1 -> Y0(1B)/1
  None2/1 -> uint_to_bus(byte)5/1
  None3/1 -> uint_to_bus(byte)6/1
  None16/1 -> uint_to_bus(byte)8/1
  None1/1 -> uint_to_bus(byte)7/1

== system Tetris/Object_Definition/T-shape (0deg) ==
  note: X
      |
      | Y
      |
      | 0
      | 1
      | 2
      | 3
      |
      | 0
      | 0
      | 1
      | 2
      |
      | 1
      |
      | 3
      |
      | 2
      |
      | 3
  None14 : Constant  OutDataTypeStr=uint8
  None15 : Constant  OutDataTypeStr=uint8
  None16 : Constant  OutDataTypeStr=uint8
  None{2,4..6} (4 alike) : Constant  Value=0  OutDataTypeStr=uint8
  None8 : Constant  Value=2  OutDataTypeStr=uint8
  uint_to_bus(byte){1..8} (8 alike) : Miscellaneous/uint_to_bus(byte)  SystemSampleTime=-1  VariantActivationTime=update diagram  Latency=0  AutoFrameSizeCalculation=off
  X0(1B) : Outport
  X1(1B) : Outport  Port=2
  X2(1B) : Outport  Port=3
  X3(1B) : Outport  Port=4
  Y0(1B) : Outport  Port=5
  Y1(1B) : Outport  Port=6
  Y2(1B) : Outport  Port=7
  Y3(1B) : Outport  Port=8
  wires:
  uint_to_bus(byte)6/1 -> Y1(1B)/1
  None16/1 -> uint_to_bus(byte)8/1
  uint_to_bus(byte)8/1 -> Y3(1B)/1
  uint_to_bus(byte)7/1 -> Y2(1B)/1
  None4/1 -> uint_to_bus(byte)7/1
  None8/1 -> uint_to_bus(byte)2/1
  None2/1 -> uint_to_bus(byte)3/1
  None5/1 -> uint_to_bus(byte)5/1
  uint_to_bus(byte)5/1 -> Y0(1B)/1
  None6/1 -> uint_to_bus(byte)6/1
  None15/1 -> uint_to_bus(byte)1/1
  None14/1 -> uint_to_bus(byte)4/1
  uint_to_bus(byte)4/1 -> X3(1B)/1
  uint_to_bus(byte)3/1 -> X0(1B)/1
  uint_to_bus(byte)1/1 -> X1(1B)/1
  uint_to_bus(byte)2/1 -> X2(1B)/1

== system Tetris/Object_Definition/T-shape (180deg) ==
  note: X
      |
      | Y
      |
      | 0
      | 1
      | 2
      | 3
      |
      | 0
      |
      | 3
      |
      | 1
      | 2
      | 1
      | 0
      |
      | 2
      |
      | 3
  None{6..8,14..15} (5 alike) : Constant  OutDataTypeStr=uint8
  None16 : Constant  Value=0  OutDataTypeStr=uint8
  None5 : Constant  Value=2  OutDataTypeStr=uint8
  None9 : Constant  Value=0  OutDataTypeStr=uint8
  uint_to_bus(byte){1..8} (8 alike) : Miscellaneous/uint_to_bus(byte)  SystemSampleTime=-1  VariantActivationTime=update diagram  Latency=0  AutoFrameSizeCalculation=off
  X0(1B) : Outport
  X1(1B) : Outport  Port=2
  X2(1B) : Outport  Port=3
  X3(1B) : Outport  Port=4
  Y0(1B) : Outport  Port=5
  Y1(1B) : Outport  Port=6
  Y2(1B) : Outport  Port=7
  Y3(1B) : Outport  Port=8
  wires:
  uint_to_bus(byte)1/1 -> X1(1B)/1
  uint_to_bus(byte)6/1 -> Y1(1B)/1
  None16/1 -> uint_to_bus(byte)8/1
  uint_to_bus(byte)8/1 -> Y3(1B)/1
  uint_to_bus(byte)7/1 -> Y2(1B)/1
  None6/1 -> uint_to_bus(byte)7/1
  uint_to_bus(byte)2/1 -> X2(1B)/1
  None9/1 -> uint_to_bus(byte)2/1
  None5/1 -> uint_to_bus(byte)3/1
  None7/1 -> uint_to_bus(byte)5/1
  uint_to_bus(byte)3/1 -> X0(1B)/1
  uint_to_bus(byte)5/1 -> Y0(1B)/1
  None8/1 -> uint_to_bus(byte)6/1
  None15/1 -> uint_to_bus(byte)1/1
  None14/1 -> uint_to_bus(byte)4/1
  uint_to_bus(byte)4/1 -> X3(1B)/1

== system Tetris/Object_Definition/T-shape (270deg) ==
  note: X
      |
      | Y
      |
      | 0
      | 1
      | 2
      | 3
      |
      | 0
      | 2
      |
      | 1
      | 1
      | 3
      |
      | 2
      | 0
      |
      | 3
  None14 : Constant  OutDataTypeStr=uint8
  None{3..4,8,15} (4 alike) : Constant  Value=0  OutDataTypeStr=uint8
  None16 : Constant  OutDataTypeStr=uint8
  None5 : Constant  Value=2  OutDataTypeStr=uint8
  None6 : Constant  OutDataTypeStr=uint8
  uint_to_bus(byte){1..8} (8 alike) : Miscellaneous/uint_to_bus(byte)  SystemSampleTime=-1  VariantActivationTime=update diagram  Latency=0  AutoFrameSizeCalculation=off
  X0(1B) : Outport
  X1(1B) : Outport  Port=2
  X2(1B) : Outport  Port=3
  X3(1B) : Outport  Port=4
  Y0(1B) : Outport  Port=5
  Y1(1B) : Outport  Port=6
  Y2(1B) : Outport  Port=7
  Y3(1B) : Outport  Port=8
  wires:
  uint_to_bus(byte)1/1 -> X1(1B)/1
  uint_to_bus(byte)6/1 -> Y1(1B)/1
  None16/1 -> uint_to_bus(byte)8/1
  uint_to_bus(byte)8/1 -> Y3(1B)/1
  uint_to_bus(byte)7/1 -> Y2(1B)/1
  None4/1 -> uint_to_bus(byte)7/1
  uint_to_bus(byte)2/1 -> X2(1B)/1
  None8/1 -> uint_to_bus(byte)2/1
  None3/1 -> uint_to_bus(byte)3/1
  None5/1 -> uint_to_bus(byte)5/1
  uint_to_bus(byte)3/1 -> X0(1B)/1
  uint_to_bus(byte)5/1 -> Y0(1B)/1
  None6/1 -> uint_to_bus(byte)6/1
  None15/1 -> uint_to_bus(byte)1/1
  None14/1 -> uint_to_bus(byte)4/1
  uint_to_bus(byte)4/1 -> X3(1B)/1

== system Tetris/Object_Definition/T-shape (90deg) ==
  note: X
      |
      | Y
      |
      | 0
      | 1
      | 2
      | 3
      |
      | 0
      |
      | 0
      |
      | 1
      | 3
      | 1
      |
      | 2
      |
      | 2
      |
      | 3
  None{1,7..8,15..16} (5 alike) : Constant  OutDataTypeStr=uint8
  None14 : Constant  Value=0  OutDataTypeStr=uint8
  None5 : Constant  Value=2  OutDataTypeStr=uint8
  None6 : Constant  Value=0  OutDataTypeStr=uint8
  uint_to_bus(byte){1..8} (8 alike) : Miscellaneous/uint_to_bus(byte)  SystemSampleTime=-1  VariantActivationTime=update diagram  Latency=0  AutoFrameSizeCalculation=off
  X0(1B) : Outport
  X1(1B) : Outport  Port=2
  X2(1B) : Outport  Port=3
  X3(1B) : Outport  Port=4
  Y0(1B) : Outport  Port=5
  Y1(1B) : Outport  Port=6
  Y2(1B) : Outport  Port=7
  Y3(1B) : Outport  Port=8
  wires:
  uint_to_bus(byte)1/1 -> X1(1B)/1
  uint_to_bus(byte)6/1 -> Y1(1B)/1
  None16/1 -> uint_to_bus(byte)8/1
  uint_to_bus(byte)8/1 -> Y3(1B)/1
  uint_to_bus(byte)7/1 -> Y2(1B)/1
  None5/1 -> uint_to_bus(byte)7/1
  uint_to_bus(byte)2/1 -> X2(1B)/1
  None8/1 -> uint_to_bus(byte)2/1
  None1/1 -> uint_to_bus(byte)3/1
  None6/1 -> uint_to_bus(byte)5/1
  uint_to_bus(byte)3/1 -> X0(1B)/1
  uint_to_bus(byte)5/1 -> Y0(1B)/1
  None7/1 -> uint_to_bus(byte)6/1
  None15/1 -> uint_to_bus(byte)1/1
  None14/1 -> uint_to_bus(byte)4/1
  uint_to_bus(byte)4/1 -> X3(1B)/1

== system Tetris/Object_Definition/Z1-shape (0deg) ==
  note: X
      |
      | Y
      |
      | 0
      | 1
      | 2
      | 3
      |
      | 0
      | 0
      | 1
      |
      | 1
      |
      | 2
      | 3
      |
      | 2
      |
      | 3
  None14 : Constant  Value=2  OutDataTypeStr=uint8
  None{8,15,19..20} (4 alike) : Constant  OutDataTypeStr=uint8
  None16 : Constant  Value=0  OutDataTypeStr=uint8
  None18 : Constant  Value=0  OutDataTypeStr=uint8
  None25 : Constant  Value=0  OutDataTypeStr=uint8
  uint_to_bus(byte){1..8} (8 alike) : Miscellaneous/uint_to_bus(byte)  SystemSampleTime=-1  VariantActivationTime=update diagram  Latency=0  AutoFrameSizeCalculation=off
  X3(1B) : Outport
  X2(1B) : Outport  Port=2
  X1(1B) : Outport  Port=3
  X0(1B) : Outport  Port=4
  Y3(1B) : Outport  Port=5
  Y2(1B) : Outport  Port=6
  Y1(1B) : Outport  Port=7
  Y0(1B) : Outport  Port=8
  wires:
  uint_to_bus(byte)3/1 -> X0(1B)/1
  uint_to_bus(byte)5/1 -> Y0(1B)/1
  uint_to_bus(byte)8/1 -> Y3(1B)/1
  uint_to_bus(byte)2/1 -> X2(1B)/1
  uint_to_bus(byte)6/1 -> Y1(1B)/1
  uint_to_bus(byte)1/1 -> X1(1B)/1
  uint_to_bus(byte)7/1 -> Y2(1B)/1
  uint_to_bus(byte)4/1 -> X3(1B)/1
  None8/1 -> uint_to_bus(byte)2/1
  None14/1 -> uint_to_bus(byte)4/1
  None15/1 -> uint_to_bus(byte)1/1
  None19/1 -> uint_to_bus(byte)7/1
  None25/1 -> uint_to_bus(byte)3/1
  None18/1 -> uint_to_bus(byte)5/1
  None16/1 -> uint_to_bus(byte)6/1
  None20/1 -> uint_to_bus(byte)8/1

== system Tetris/Object_Definition/Z1-shape (90deg) ==
  note: X
      |
      | Y
      |
      | 0
      | 1
      | 2
      | 3
      |
      | 0
      |
      | 0
      |
      | 1
      | 2
      | 1
      |
      | 2
      | 3
      |
      | 3
  None1 : Constant  Value=0  OutDataTypeStr=uint8
  None2 : Constant  Value=0  OutDataTypeStr=uint8
  None{3..4,6,25} (4 alike) : Constant  OutDataTypeStr=uint8
  None5 : Constant  Value=0  OutDataTypeStr=uint8
  None7 : Constant  Value=2  OutDataTypeStr=uint8
  uint_to_bus(byte){1..8} (8 alike) : Miscellaneous/uint_to_bus(byte)  SystemSampleTime=-1  VariantActivationTime=update diagram  Latency=0  AutoFrameSizeCalculation=off
  X3(1B) : Outport
  X2(1B) : Outport  Port=2
  X1(1B) : Outport  Port=3
  X0(1B) : Outport  Port=4
  Y3(1B) : Outport  Port=5
  Y2(1B) : Outport  Port=6
  Y1(1B) : Outport  Port=7
  Y0(1B) : Outport  Port=8
  wires:
  uint_to_bus(byte)3/1 -> X0(1B)/1
  None25/1 -> uint_to_bus(byte)3/1
  None4/1 -> uint_to_bus(byte)6/1
  None5/1 -> uint_to_bus(byte)5/1
  None1/1 -> uint_to_bus(byte)2/1
  None7/1 -> uint_to_bus(byte)8/1
  uint_to_bus(byte)4/1 -> X3(1B)/1
  None2/1 -> uint_to_bus(byte)4/1
  uint_to_bus(byte)2/1 -> X2(1B)/1
  uint_to_bus(byte)1/1 -> X1(1B)/1
  uint_to_bus(byte)7/1 -> Y2(1B)/1
  None6/1 -> uint_to_bus(byte)7/1
  uint_to_bus(byte)6/1 -> Y1(1B)/1
  uint_to_bus(byte)5/1 -> Y0(1B)/1
  None3/1 -> uint_to_bus(byte)1/1
  uint_to_bus(byte)8/1 -> Y3(1B)/1

== system Tetris/Object_Definition/Z2-shape (0deg) ==
  note: X
      |
      | Y
      |
      | 0
      | 1
      | 2
      | 3
      |
      | 0
      |
      | 1
      | 0
      |
      | 1
      | 3
      | 2
      |
      | 2
      |
      | 3
  None14 : Constant  Value=0  OutDataTypeStr=uint8
  None{4,8,15..16} (4 alike) : Constant  OutDataTypeStr=uint8
  None2 : Constant  Value=2  OutDataTypeStr=uint8
  None5 : Constant  Value=0  OutDataTypeStr=uint8
  None6 : Constant  Value=0  OutDataTypeStr=uint8
  uint_to_bus(byte){1..8} (8 alike) : Miscellaneous/uint_to_bus(byte)  SystemSampleTime=-1  VariantActivationTime=update diagram  Latency=0  AutoFrameSizeCalculation=off
  X0(1B) : Outport
  X1(1B) : Outport  Port=2
  X2(1B) : Outport  Port=3
  X3(1B) : Outport  Port=4
  Y0(1B) : Outport  Port=5
  Y1(1B) : Outport  Port=6
  Y2(1B) : Outport  Port=7
  Y3(1B) : Outport  Port=8
  wires:
  uint_to_bus(byte)2/1 -> X2(1B)/1
  uint_to_bus(byte)3/1 -> X0(1B)/1
  uint_to_bus(byte)7/1 -> Y2(1B)/1
  None5/1 -> uint_to_bus(byte)5/1
  None6/1 -> uint_to_bus(byte)6/1
  uint_to_bus(byte)5/1 -> Y0(1B)/1
  None2/1 -> uint_to_bus(byte)3/1
  None8/1 -> uint_to_bus(byte)2/1
  None15/1 -> uint_to_bus(byte)1/1
  None4/1 -> uint_to_bus(byte)7/1
  uint_to_bus(byte)8/1 -> Y3(1B)/1
  None16/1 -> uint_to_bus(byte)8/1
  uint_to_bus(byte)1/1 -> X1(1B)/1
  uint_to_bus(byte)6/1 -> Y1(1B)/1
  None14/1 -> uint_to_bus(byte)4/1
  uint_to_bus(byte)4/1 -> X3(1B)/1

== system Tetris/Object_Definition/Z2-shape (90deg) ==
  note: X
      |
      | Y
      |
      | 0
      | 1
      | 2
      | 3
      |
      | 0
      | 0
      |
      | 1
      | 1
      | 2
      |
      | 2
      |
      | 3
      |
      | 3
  None{4,6,8,14} (4 alike) : Constant  OutDataTypeStr=uint8
  None15 : Constant  Value=0  OutDataTypeStr=uint8
  None16 : Constant  Value=2  OutDataTypeStr=uint8
  None3 : Constant  Value=0  OutDataTypeStr=uint8
  None5 : Constant  Value=0  OutDataTypeStr=uint8
  uint_to_bus(byte){1..8} (8 alike) : Miscellaneous/uint_to_bus(byte)  SystemSampleTime=-1  VariantActivationTime=update diagram  Latency=0  AutoFrameSizeCalculation=off
  X0(1B) : Outport
  X1(1B) : Outport  Port=2
  X2(1B) : Outport  Port=3
  X3(1B) : Outport  Port=4
  Y0(1B) : Outport  Port=5
  Y1(1B) : Outport  Port=6
  Y2(1B) : Outport  Port=7
  Y3(1B) : Outport  Port=8
  wires:
  uint_to_bus(byte)1/1 -> X1(1B)/1
  uint_to_bus(byte)6/1 -> Y1(1B)/1
  None16/1 -> uint_to_bus(byte)8/1
  uint_to_bus(byte)8/1 -> Y3(1B)/1
  uint_to_bus(byte)7/1 -> Y2(1B)/1
  None4/1 -> uint_to_bus(byte)7/1
  uint_to_bus(byte)2/1 -> X2(1B)/1
  None8/1 -> uint_to_bus(byte)2/1
  None3/1 -> uint_to_bus(byte)3/1
  None5/1 -> uint_to_bus(byte)5/1
  uint_to_bus(byte)3/1 -> X0(1B)/1
  uint_to_bus(byte)5/1 -> Y0(1B)/1
  None6/1 -> uint_to_bus(byte)6/1
  None15/1 -> uint_to_bus(byte)1/1
  None14/1 -> uint_to_bus(byte)4/1
  uint_to_bus(byte)4/1 -> X3(1B)/1
